simulink model "three_phase_induction_motor_speed_controller"  (R2020b)
settings: Solver=FixedStepAuto  StartTime=0.0  StopTime=200  RelTol=1e-3
undefined symbols (not defined in the file): Continuous, gcbh, J, Lm, Lr, Ls, p, Rr, Rs, sps, sps_rtmsupport, spsTriangleGeneratorModel
libraries: powerlib x13, simulink x5, pid_lib x2
settings Model: Creator=Vibhusha  LastModifiedBy=Vibhusha
settings DataIOCC: ReturnWorkspaceOutputs=off
settings DebuggingCC: ArithmeticOperatorsInVariantConditions=warning
settings SFSimCC: SimUseLocalCustomCode=off  CustomCodeUndefinedFunction=UseInterfaceOnly
settings RTWCC: RTWUseLocalCustomCode=off

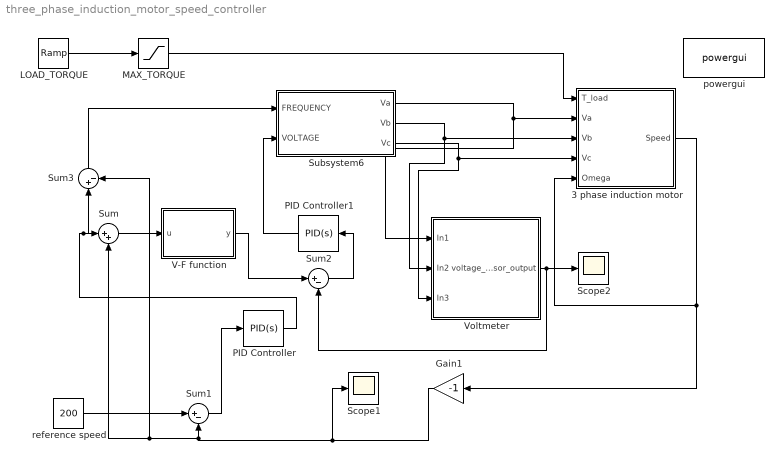
== system three_phase_induction_motor_speed_controller ==
  3 phase induction motor : Subsystem
  Gain1 : Gain  Gain=-1
  LOAD_TORQUE : simulink/Sources/Ramp  slope=0.1  start=0  InitialOutput=0
  MAX_TORQUE : Saturate  UpperLimit=5  LowerLimit=0
  PID Controller : pid_lib/PID Controller  Controller=PID  Form=Parallel  TimeDomain=Continuous-time  UseExternalTs=off  SampleTime=-1  IntegratorMethod=Forward Euler  FilterMethod=Forward Euler  ControllerParametersSource=internal  P=400  I=0.00001  D=0.0001  UseFilter=on  N=50  TunerSelectOption=Transfer Function Based (PID Tuner App)  InitialConditionSource=internal  InitialConditionForIntegrator=0  InitialConditionForFilter=0  DifferentiatorICPrevScaledInput=0  ExternalReset=none  TrackingMode=off  Kt=1  LimitOutput=on  SatLimitsSource=internal  UpperSaturationLimit=4000  LowerSaturationLimit=0  LinearizeAsGain=on  AntiWindupMode=none  Kb=1  POutMin=[]  POutMax=[]  IOutMin=[]  IOutMax=[]  DOutMin=[]  DOutMax=[]  NOutMin=[]  NOutMax=[]  SumOutMin=[]  SumOutMax=[]  SaturationOutMin=[]  SaturationOutMax=[]  PParamMin=[]  PParamMax=[]  IParamMin=[]  IParamMax=[]  DParamMin=[]  DParamMax=[]  NParamMin=[]  NParamMax=[]  KbParamMin=[]  KbParamMax=[]  KtParamMin=[]  KtParamMax=[]  KbOutMin=[]  KbOutMax=[]  KtOutMin=[]  KtOutMax=[]  IntegratorOutMin=[]  IntegratorOutMax=[]  FilterOutMin=[]  FilterOutMax=[]  SumI1OutMin=[]  SumI1OutMax=[]  SumI2OutMin=[]  SumI2OutMax=[]  SumI3OutMin=[]  SumI3OutMax=[]  SumI4OutMin=[]  SumI4OutMax=[]  SumDOutMin=[]  SumDOutMax=[]  DifferentiatorOutMin=[]  DifferentiatorOutMax=[]  FilterDiffOutCoefMin=[]  FilterDiffOutCoefMax=[]  ReciprocalOutMin=[]  ReciprocalOutMax=[]  SumDenOutMin=[]  SumDenOutMax=[]  SumNumOutMin=[]  SumNumOutMax=[]  DivideOutMin=[]  DivideOutMax=[]  UdiffTsProdOutMin=[]  UdiffTsProdOutMax=[]  NTsProdOutMin=[]  NTsProdOutMax=[]  UintegralTsProdOutMin=[]  UintegralTsProdOutMax=[]  UngainTsProdOutMin=[]  UngainTsProdOutMax=[]  IntegratorContinuousStateAttributes=''  IntegratorStateMustResolveToSignalObject=off  IntegratorRTWStateStorageClass=Auto  FilterContinuousStateAttributes=''  FilterStateMustResolveToSignalObject=off  FilterRTWStateStorageClass=Auto  ParallelPVariant=InternalParameters  IdealPVariant=Disabled  IVariant=InternalParameters  DVariant=InternalParameters  IntegratorVariant=Continuous  SatVariant=Enabled  AWVariant=Passthrough  PCopyVariant=Disabled  TRVariant=Disabled  FdbkBlocksVariant=Forward  IdealPFdbkVariant=Disabled  SatFdbkVariant=Disabled  DerivativeFilterVariant=ContFilter  NVariant=InternalParameters  NCopyVariant=Disabled  FilterICVariant=InternalICsFilter  IntegratorICVariant=InternalICs  ExternalResetVariant=Disabled  TRSumVariant=Passthrough  SumFdbkVariant=Disabled  SumVariant=Sum_PID  TsampFilterVariant=InternalTs  TsampNgainVariant=Passthrough  TsampIntegralVariant=Passthrough  ExternalSaturationOutDataTypeStr=Inherit: Same as second input
  PID Controller1 : pid_lib/PID Controller  Controller=PID  Form=Parallel  TimeDomain=Continuous-time  UseExternalTs=off  SampleTime=-1  IntegratorMethod=Forward Euler  FilterMethod=Forward Euler  ControllerParametersSource=internal  P=400  I=0.00001  D=0  UseFilter=on  N=50  TunerSelectOption=Transfer Function Based (PID Tuner App)  InitialConditionSource=internal  InitialConditionForIntegrator=0  InitialConditionForFilter=0  DifferentiatorICPrevScaledInput=0  ExternalReset=none  TrackingMode=off  Kt=1  LimitOutput=on  SatLimitsSource=internal  UpperSaturationLimit=inf  LowerSaturationLimit=1  LinearizeAsGain=on  AntiWindupMode=none  Kb=1  POutMin=[]  POutMax=[]  IOutMin=[]  IOutMax=[]  DOutMin=[]  DOutMax=[]  NOutMin=[]  NOutMax=[]  SumOutMin=[]  SumOutMax=[]  SaturationOutMin=[]  SaturationOutMax=[]  PParamMin=[]  PParamMax=[]  IParamMin=[]  IParamMax=[]  DParamMin=[]  DParamMax=[]  NParamMin=[]  NParamMax=[]  KbParamMin=[]  KbParamMax=[]  KtParamMin=[]  KtParamMax=[]  KbOutMin=[]  KbOutMax=[]  KtOutMin=[]  KtOutMax=[]  IntegratorOutMin=[]  IntegratorOutMax=[]  FilterOutMin=[]  FilterOutMax=[]  SumI1OutMin=[]  SumI1OutMax=[]  SumI2OutMin=[]  SumI2OutMax=[]  SumI3OutMin=[]  SumI3OutMax=[]  SumI4OutMin=[]  SumI4OutMax=[]  SumDOutMin=[]  SumDOutMax=[]  DifferentiatorOutMin=[]  DifferentiatorOutMax=[]  FilterDiffOutCoefMin=[]  FilterDiffOutCoefMax=[]  ReciprocalOutMin=[]  ReciprocalOutMax=[]  SumDenOutMin=[]  SumDenOutMax=[]  SumNumOutMin=[]  SumNumOutMax=[]  DivideOutMin=[]  DivideOutMax=[]  UdiffTsProdOutMin=[]  UdiffTsProdOutMax=[]  NTsProdOutMin=[]  NTsProdOutMax=[]  UintegralTsProdOutMin=[]  UintegralTsProdOutMax=[]  UngainTsProdOutMin=[]  UngainTsProdOutMax=[]  IntegratorContinuousStateAttributes=''  IntegratorStateMustResolveToSignalObject=off  IntegratorRTWStateStorageClass=Auto  FilterContinuousStateAttributes=''  FilterStateMustResolveToSignalObject=off  FilterRTWStateStorageClass=Auto  ParallelPVariant=InternalParameters  IdealPVariant=Disabled  IVariant=InternalParameters  DVariant=InternalParameters  IntegratorVariant=Continuous  SatVariant=Enabled  AWVariant=Passthrough  PCopyVariant=Disabled  TRVariant=Disabled  FdbkBlocksVariant=Forward  IdealPFdbkVariant=Disabled  SatFdbkVariant=Disabled  DerivativeFilterVariant=ContFilter  NVariant=InternalParameters  NCopyVariant=Disabled  FilterICVariant=InternalICsFilter  IntegratorICVariant=InternalICs  ExternalResetVariant=Disabled  TRSumVariant=Passthrough  SumFdbkVariant=Disabled  SumVariant=Sum_PID  TsampFilterVariant=InternalTs  TsampNgainVariant=Passthrough  TsampIntegralVariant=Passthrough  ExternalSaturationOutDataTypeStr=Inherit: Same as second input
  Scope1 : Scope
  Scope2 : Scope
  Subsystem6 : Subsystem
  Sum : Sum  Inputs=|++
  Sum1 : Sum  Inputs=|+-
  Sum2 : Sum  Inputs=|+-
  Sum3 : Sum  Inputs=|+-
  V-F function : MATLAB Function  TreatAsAtomicUnit=on
  Voltmeter : Subsystem
  powergui : powerlib/powergui  Priority=1  SimulationMode=Continuous  SampleTime=50e-6  frequency=60  Iterations=50  frequencyindice=0  Pbase=100e6  ErrMax=1e-4  UnitsV=kV  UnitsW=MW  buscounter=0  FunctionMessages=off  echomessages=off  EnableUseOfTLC=off  CurrentSourceSwitches=off  DisableSnubberDevices=off  DisableRonSwitches=off  DisableVfSwitches=off  DisplayEquations=off  AutomaticDiscreteSolvers=off  SolverType=Tustin/Backward Euler (TBE)  Interpol=off  ExternalGateDelay=off  methode=off  Ts=100  x0status=blocks  SPID=on  SwTol=0  HookPort=off  NonlinearTolerance=1e-4  nMaxIteration=100  ContinueOnMaxIteration=off  RestoreLinks=warning  ResistiveCurrentMeasurement=off  Frange=[0:2:500]  Ylog=off  Xlog=on  ShowGrid=off  save=off  variable=ZData  structure=0  ZoomFFT=off  StartTime=0.0  cycles=1  DisplayStyle=1  fundamental=60  FreqAxis=off  MaxFrequency=1000  frequencyindicesteady=1  RmsSteady=1  display=off
  reference speed : Constant  Value=200
  wires:
  Subsystem6/1(Va) -> Voltmeter/1(In1), 3 phase induction motor/2(Va)
  Subsystem6/2(Vb) -> Voltmeter/2(In2), 3 phase induction motor/3(Vb)
  Subsystem6/3(Vc) -> Voltmeter/3(In3), 3 phase induction motor/4(Vc)
  reference speed/1 -> Sum1/1
  Sum1/1 -> PID Controller/1
  Gain1/1 -> Sum3/2, Sum/2, Sum1/2, Scope1/1
  V-F function/1(y) -> Sum2/1
  Sum2/1 -> PID Controller1/1
  PID Controller1/1 -> Subsystem6/2(VOLTAGE)
  PID Controller/1 -> Sum3/1, Sum/1
  LOAD_TORQUE/1 -> MAX_TORQUE/1
  Voltmeter/1(voltage_sensor_output) -> Scope2/1, Sum2/2
  3 phase induction motor/1(Speed) -> Gain1/1, 3 phase induction motor/5(Omega)
  MAX_TORQUE/1 -> 3 phase induction motor/1(T_load)
  Sum/1 -> V-F function/1(u)
  Sum3/1 -> Subsystem6/1(FREQUENCY)

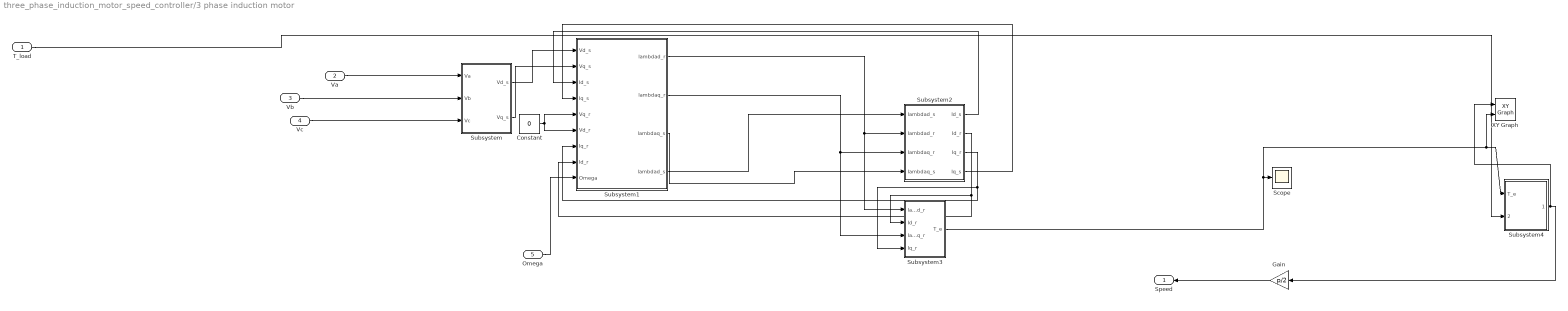
== system three_phase_induction_motor_speed_controller/3 phase induction motor ==
  T_load : Inport
  Va : Inport  Port=2
  Vb : Inport  Port=3
  Vc : Inport  Port=4
  Omega : Inport  Port=5
  Constant : Constant  Value=0
  Gain : Gain  Gain=p/2
  Scope : Scope
  Subsystem : Subsystem
  Subsystem1 : Subsystem
  Subsystem2 : Subsystem
  Subsystem3 : Subsystem
  Subsystem4 : Subsystem
  XY Graph : simulink/Sinks/XY Graph  xmin=-1  xmax=1  ymin=-1  ymax=1  st=-1
  Speed : Outport
  wires:
  Subsystem2/3(Iq_r) -> Subsystem3/4(Iq_r), Subsystem1/7(Iq_r)
  Subsystem3/1(T_e) -> XY Graph/2, Subsystem4/1(T_e), Scope/1
  Subsystem2/2(Id_r) -> Subsystem1/8(Id_r), Subsystem3/2(Id_r)
  Subsystem2/1(Id_s) -> Subsystem1/3(Id_s)
  Subsystem2/4(Iq_s) -> Subsystem1/4(Iq_s)
  Vc/1 -> Subsystem/3(Vc)
  Va/1 -> Subsystem/1(Va)
  Subsystem1/1(lambdad_r) -> Subsystem2/2(Iambdad_r), Subsystem3/1(lambdad_r)
  Subsystem1/3(lambdaq_s) -> Subsystem2/4(Iambdaq_s)
  Constant/1 -> Subsystem1/6(Vd_r), Subsystem1/5(Vq_r)
  Subsystem/2(Vq_s) -> Subsystem1/2(Vq_s)
  Omega/1 -> Subsystem1/9(Omega)
  T_load/1 -> Subsystem4/2(T_load)
  Subsystem/1(Vd_s) -> Subsystem1/1(Vd_s)
  Subsystem1/2(lambdaq_r) -> Subsystem3/3(Iambdaq_r), Subsystem2/3(Iambdaq_r)
  Subsystem4/1(W_mech) -> XY Graph/1, Gain/1
  Vb/1 -> Subsystem/2(Vb)
  Subsystem1/4(lambdad_s) -> Subsystem2/1(Iambdad_s)
  Gain/1 -> Speed/1

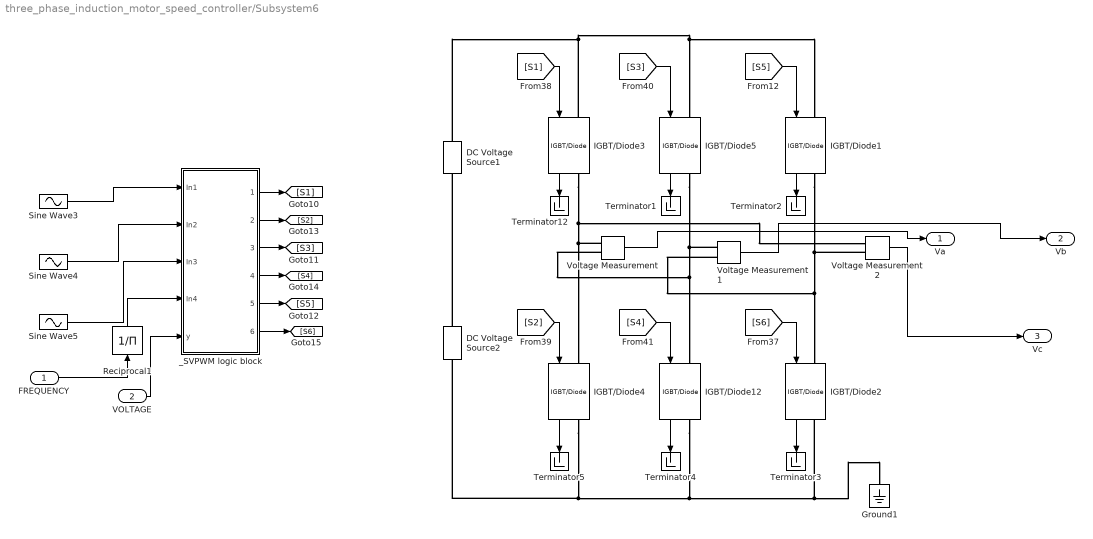
== system three_phase_induction_motor_speed_controller/Subsystem6 ==
  FREQUENCY : Inport
  VOLTAGE : Inport  Port=2
  DC Voltage Source1 : powerlib/Electrical Sources/DC Voltage Source  Amplitude=125  Measurements=None
  DC Voltage Source2 : powerlib/Electrical Sources/DC Voltage Source  Amplitude=125  Measurements=None
  Ground1 : powerlib/Elements/Ground  LConnTagsString=a
  IGBT/Diode{1..5,12} (6 alike) : powerlib/Power Electronics/IGBT//Diode  Ron=1e-3  Rs=1e5  Cs=inf  Measurements=on
  Reciprocal1 : Product  Inputs=/
  Sine Wave3 : Sin  Frequency=50*2*pi  SampleTime=0
  Sine Wave4 : Sin  Frequency=50*2*pi  Phase=pi*(-2/3)  SampleTime=0
  Sine Wave5 : Sin  Frequency=50*2*pi  Phase=pi*(2/3)  SampleTime=0
  Terminator{1..5,12} (6 alike) : Terminator
  Voltage Measurement : powerlib/Measurements/Voltage Measurement  PhasorSimulation=off  OutputType=Complex  PSBequivalent=0
  Voltage Measurement1 : powerlib/Measurements/Voltage Measurement  PhasorSimulation=off  OutputType=Complex  PSBequivalent=0
  Voltage Measurement2 : powerlib/Measurements/Voltage Measurement  PhasorSimulation=off  OutputType=Complex  PSBequivalent=0
  _SVPWM logic block : Subsystem
  Va : Outport
  Vb : Outport  Port=2
  Vc : Outport  Port=3
  wires:
  Sine Wave5/1 -> _SVPWM logic block/3(In3)
  IGBT/Diode3/1 -> Terminator12/1
  [S1] -> IGBT/Diode3/1
  _SVPWM logic block/6(6) -> [S6]
  Sine Wave4/1 -> _SVPWM logic block/2(In2)
  _SVPWM logic block/1(1) -> [S1]
  IGBT/Diode1/1 -> Terminator2/1
  IGBT/Diode2/1 -> Terminator3/1
  IGBT/Diode4/1 -> Terminator5/1
  IGBT/Diode5/1 -> Terminator1/1
  [S2] -> IGBT/Diode4/1
  _SVPWM logic block/4(4) -> [S4]
  _SVPWM logic block/5(5) -> [S5]
  [S3] -> IGBT/Diode5/1
  [S6] -> IGBT/Diode2/1
  Sine Wave3/1 -> _SVPWM logic block/1(In1)
  [S4] -> IGBT/Diode12/1
  _SVPWM logic block/3(3) -> [S3]
  [S5] -> IGBT/Diode1/1
  IGBT/Diode12/1 -> Terminator4/1
  _SVPWM logic block/2(2) -> [S2]
  Voltage Measurement/1 -> Va/1
  Voltage Measurement1/1 -> Vb/1
  Voltage Measurement2/1 -> Vc/1
  FREQUENCY/1 -> Reciprocal1/1
  VOLTAGE/1 -> _SVPWM logic block/5(y)
  Reciprocal1/1 -> _SVPWM logic block/4(In4)
  connections:
  DC Voltage Source2/RConn1 -- DC Voltage Source1/LConn1
  IGBT/Diode1/RConn1 -- Voltage Measurement1/LConn2 -- IGBT/Diode2/LConn1 -- Voltage Measurement2/LConn2
  IGBT/Diode4/RConn1 -- IGBT/Diode12/RConn1 -- Ground1/LConn1 -- IGBT/Diode2/RConn1 -- DC Voltage Source2/LConn1
  IGBT/Diode5/RConn1 -- Voltage Measurement1/LConn1 -- Voltage Measurement/LConn2 -- IGBT/Diode12/LConn1
  IGBT/Diode3/RConn1 -- IGBT/Diode4/LConn1 -- Voltage Measurement/LConn1 -- Voltage Measurement2/LConn1
  IGBT/Diode3/LConn1 -- IGBT/Diode1/LConn1 -- IGBT/Diode5/LConn1 -- DC Voltage Source1/RConn1

== system three_phase_induction_motor_speed_controller/Voltmeter ==
  In1 : Inport
  In2 : Inport  Port=2
  In3 : Inport  Port=3
  Abs : Abs
  Abs1 : Abs
  Abs2 : Abs
  Sum : Sum  Inputs=|+++
  voltage_sensor_output : Outport
  wires:
  In1/1 -> Abs2/1
  Abs2/1 -> Sum/1
  In3/1 -> Abs1/1
  Abs1/1 -> Sum/3
  In2/1 -> Abs/1
  Abs/1 -> Sum/2
  Sum/1 -> voltage_sensor_output/1

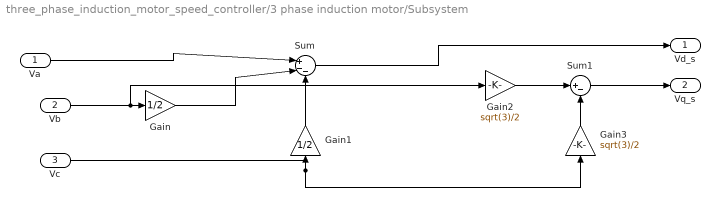
== system three_phase_induction_motor_speed_controller/3 phase induction motor/Subsystem ==
  Va : Inport
  Vb : Inport  Port=2
  Vc : Inport  Port=3
  Gain : Gain  Gain=1/2
  Gain1 : Gain  Gain=1/2
  Gain2 : Gain  Gain=sqrt(3)/2
  Gain3 : Gain  Gain=sqrt(3)/2
  Sum : Sum  Inputs=|+--
  Sum1 : Sum  Inputs=|+-
  Vd_s : Outport  VectorParamsAs1DForOutWhenUnconnected=off
  Vq_s : Outport  Port=2  VectorParamsAs1DForOutWhenUnconnected=off
  wires:
  Vc/1 -> Gain3/1, Gain1/1
  Sum1/1 -> Vq_s/1
  Vb/1 -> Gain2/1, Gain/1
  Gain2/1 -> Sum1/1
  Gain3/1 -> Sum1/2
  Gain/1 -> Sum/2
  Va/1 -> Sum/1
  Gain1/1 -> Sum/3
  Sum/1 -> Vd_s/1

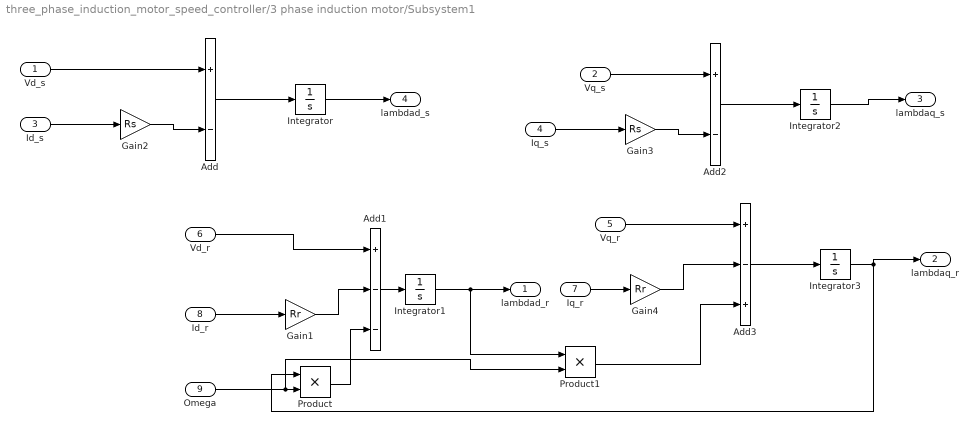
== system three_phase_induction_motor_speed_controller/3 phase induction motor/Subsystem1 ==
  Vd_s : Inport
  Vq_s : Inport  Port=2
  Id_s : Inport  Port=3
  Iq_s : Inport  Port=4
  Vq_r : Inport  Port=5
  Vd_r : Inport  Port=6
  Iq_r : Inport  Port=7
  Id_r : Inport  Port=8
  Omega : Inport  Port=9
  Add : Sum  Inputs=+-
  Add1 : Sum  Inputs=+--
  Add2 : Sum  Inputs=+-
  Add3 : Sum  Inputs=+-+
  Gain1 : Gain  Gain=Rr
  Gain2 : Gain  Gain=Rs
  Gain3 : Gain  Gain=Rs
  Gain4 : Gain  Gain=Rr
  Integrator{,1..3} (4 alike) : Integrator
  Product : Product
  Product1 : Product
  lambdad_r : Outport  VectorParamsAs1DForOutWhenUnconnected=off
  lambdaq_r : Outport  Port=2  VectorParamsAs1DForOutWhenUnconnected=off
  lambdaq_s : Outport  Port=3  VectorParamsAs1DForOutWhenUnconnected=off
  lambdad_s : Outport  Port=4  VectorParamsAs1DForOutWhenUnconnected=off
  wires:
  Integrator/1 -> lambdad_s/1
  Gain2/1 -> Add/2
  Integrator3/1 -> lambdaq_r/1, Product/1
  Vd_r/1 -> Add1/1
  Id_r/1 -> Gain1/1
  Add/1 -> Integrator/1
  Integrator2/1 -> lambdaq_s/1
  Id_s/1 -> Gain2/1
  Product/1 -> Add1/3
  Gain3/1 -> Add2/2
  Omega/1 -> Product1/2, Product/2
  Add2/1 -> Integrator2/1
  Integrator1/1 -> lambdad_r/1, Product1/1
  Gain1/1 -> Add1/2
  Vq_r/1 -> Add3/1
  Iq_r/1 -> Gain4/1
  Add1/1 -> Integrator1/1
  Vq_s/1 -> Add2/1
  Iq_s/1 -> Gain3/1
  Product1/1 -> Add3/3
  Add3/1 -> Integrator3/1
  Gain4/1 -> Add3/2
  Vd_s/1 -> Add/1

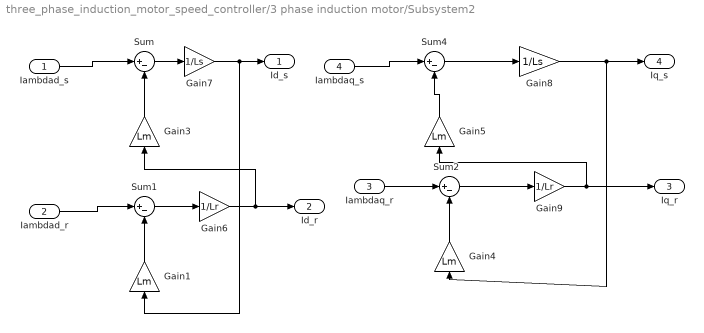
== system three_phase_induction_motor_speed_controller/3 phase induction motor/Subsystem2 ==
  Iambdad_s : Inport
  Iambdad_r : Inport  Port=2
  Iambdaq_r : Inport  Port=3
  Iambdaq_s : Inport  Port=4
  Gain{1,3..5} (4 alike) : Gain  Gain=Lm
  Gain6 : Gain  Gain=1/Lr
  Gain7 : Gain  Gain=1/Ls
  Gain8 : Gain  Gain=1/Ls
  Gain9 : Gain  Gain=1/Lr
  Sum{,1..2,4} (4 alike) : Sum  Inputs=|+-
  Id_s : Outport  VectorParamsAs1DForOutWhenUnconnected=off
  Id_r : Outport  Port=2  VectorParamsAs1DForOutWhenUnconnected=off
  Iq_r : Outport  Port=3  VectorParamsAs1DForOutWhenUnconnected=off
  Iq_s : Outport  Port=4  VectorParamsAs1DForOutWhenUnconnected=off
  wires:
  Sum/1 -> Gain7/1
  Gain6/1 -> Id_r/1, Gain3/1
  Iambdad_s/1 -> Sum/1
  Gain4/1 -> Sum2/2
  Gain8/1 -> Iq_s/1, Gain4/1
  Sum2/1 -> Gain9/1
  Gain5/1 -> Sum4/2
  Gain3/1 -> Sum/2
  Gain9/1 -> Iq_r/1, Gain5/1
  Gain7/1 -> Id_s/1, Gain1/1
  Iambdad_r/1 -> Sum1/1
  Iambdaq_r/1 -> Sum2/1
  Gain1/1 -> Sum1/2
  Sum1/1 -> Gain6/1
  Sum4/1 -> Gain8/1
  Iambdaq_s/1 -> Sum4/1

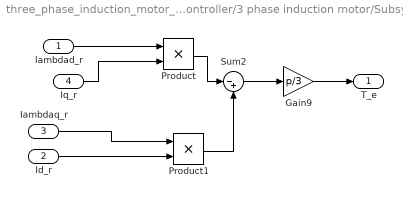
== system three_phase_induction_motor_speed_controller/3 phase induction motor/Subsystem3 ==
  lambdad_r : Inport
  Id_r : Inport  Port=2
  Iambdaq_r : Inport  Port=3
  Iq_r : Inport  Port=4
  Gain9 : Gain  Gain=p/3
  Product : Product
  Product1 : Product
  Sum2 : Sum  Inputs=|-+
  T_e : Outport  VectorParamsAs1DForOutWhenUnconnected=off
  wires:
  Product1/1 -> Sum2/2
  Product/1 -> Sum2/1
  Sum2/1 -> Gain9/1
  Gain9/1 -> T_e/1
  Iambdaq_r/1 -> Product1/1
  Iq_r/1 -> Product/2
  lambdad_r/1 -> Product/1
  Id_r/1 -> Product1/2

== system three_phase_induction_motor_speed_controller/3 phase induction motor/Subsystem4 ==
  T_e : Inport
  T_load : Inport  Port=2
  Gain : Gain  Gain=1/J
  Gain1 : Gain  Gain=2/p
  Integrator : Integrator
  Sum : Sum  Inputs=|+-
  W_mech : Outport  VectorParamsAs1DForOutWhenUnconnected=off
  wires:
  Sum/1 -> Gain/1
  T_load/1 -> Sum/2
  Integrator/1 -> Gain1/1
  Gain/1 -> Integrator/1
  Gain1/1 -> W_mech/1
  T_e/1 -> Sum/1

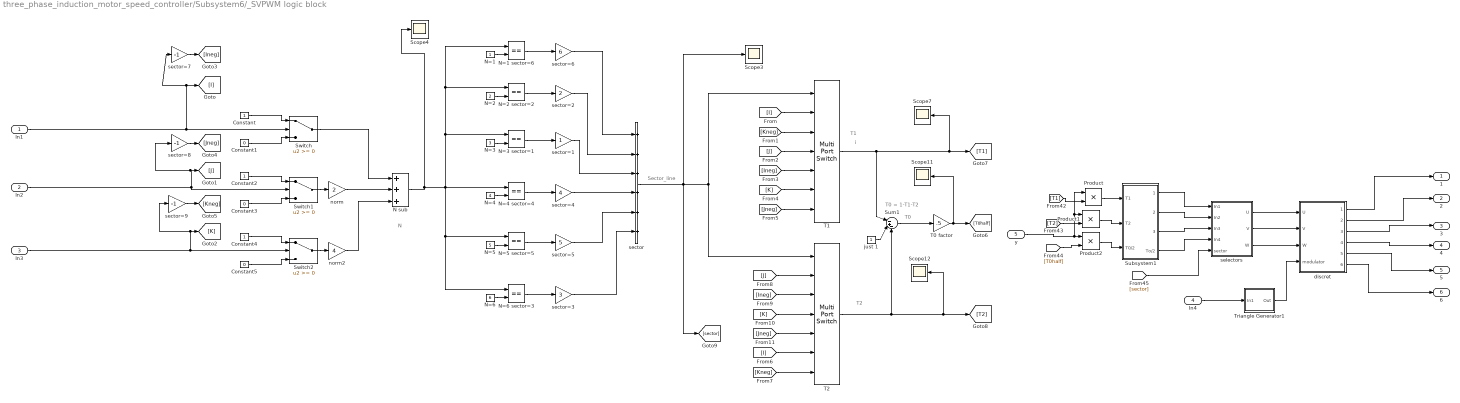
== system three_phase_induction_motor_speed_controller/Subsystem6/_SVPWM logic block ==
  note: T0
  note: T0 = 1-T1-T2
  note: T2
  note: T1
  note: i
  note: Sector_line
  note: N
  In1 : Inport
  In2 : Inport  Port=2
  In3 : Inport  Port=3
  In4 : Inport  Port=4
  y : Inport  Port=5
  Constant : Constant
  Constant1 : Constant  Value=0
  Constant2 : Constant
  Constant3 : Constant  Value=0
  Constant4 : Constant
  Constant5 : Constant  Value=0
  N sub : Sum  Inputs=+++
  N=1 : Constant
  N=1 sector=6 : RelationalOperator  Operator===  OutDataTypeStr=boolean  RndMeth=Nearest
  N=2 : Constant  Value=2
  N=2 sector=2 : RelationalOperator  Operator===  OutDataTypeStr=boolean  RndMeth=Nearest
  N=3 : Constant  Value=3
  N=3 sector=1 : RelationalOperator  Operator===  OutDataTypeStr=boolean  RndMeth=Nearest
  N=4 : Constant  Value=4
  N=4 sector=4 : RelationalOperator  Operator===  OutDataTypeStr=boolean  RndMeth=Nearest
  N=5 : Constant  Value=5
  N=5 sector=5 : RelationalOperator  Operator===  OutDataTypeStr=boolean  RndMeth=Nearest
  N=6 : Constant  Value=6
  N=6 sector=3 : RelationalOperator  Operator===  OutDataTypeStr=boolean  RndMeth=Nearest
  Product : Product
  Product1 : Product
  Product2 : Product
  Scope{3..4,7,11..12} (5 alike) : Scope
  Subsystem1 : Subsystem
  Sum1 : Sum  Inputs=|-+-
  Switch : Switch
  Switch1 : Switch
  Switch2 : Switch
  T0 factor : Gain  Gain=.5
  T1 : MultiPortSwitch  DataPortOrder=Specify indices  Inputs=4  DataPortIndices={1,2,3,4,5,6}
  T2 : MultiPortSwitch  DataPortOrder=Specify indices  Inputs=4  DataPortIndices={1,2,3,4,5,6}
  Triangle Generator1 : Subsystem  AncestorBlock=|  DialogController=POWERSYS.PowerSysDialog  LoadFcn=sps_rtmsupport('LoadFcn', gcbh);  StartFcn=sps_rtmsupport('StartFcn', gcbh);  StopFcn=sps_rtmsupport('StopFcn', gcbh);  mask(Triangle Generator){Freq=100, Phase=180, Ts=0}
      | powerlib_meascontrol/Pulse & Signal
      | Generators/Triangle
      | Generator
      mask prompts: Freq "Frequency (Hz):"; Phase "Phase (degrees):"; Ts "Sample time:"
      mask help: Generate a symmetrical triangle wave with peak amplitude of +/- 1.
      mask init:
      | block = gcb;
      | [WantBlockChoice,Ts,sps] = powericon('TriangleGeneratorInit',block,Phase,Freq,Ts);
      | powericon('SetInternalModels','set',block,WantBlockChoice);
      settings: CopyFcn=sps_rtmsupport('CopyFcn', gcbh);  DeleteFcn=sps_rtmsupport('DeleteFcn', gcbh);  UndoDeleteFcn=sps_rtmsupport('UndoDeleteFcn', gcbh);  ModelCloseFcn=sps_rtmsupport('ModelCloseFcn', gcbh);  PreSaveFcn=sps_rtmsupport('PreSaveFcn', gcbh);  PostSaveFcn=sps_rtmsupport('PostSaveFcn', gcbh);  NameChangeFcn=sps_rtmsupport('NameChangeFcn', gcbh);  PreCopyFcn=sps_rtmsupport('PreCopyFcn', gcbh);  OpenFcn=sps_rtmsupport('OpenFcn', gcbh, []);  CloseFcn=sps_rtmsupport('CloseFcn', gcbh);  PreDeleteFcn=sps_rtmsupport('PreDeleteFcn', gcbh);
      mask Help: helpview(psbhelp);
      mask Display: plot([sps.time sps.time+sps.time(end)],repmat(sps.Out,1,2))
  discret : Subsystem
  just 1 : Constant
  norm : Gain  Gain=2
  norm2 : Gain  Gain=4
  sector : Sum  Inputs=++++++
  sector=1 : Gain
  sector=2 : Gain  Gain=2
  sector=3 : Gain  Gain=3
  sector=4 : Gain  Gain=4
  sector=5 : Gain  Gain=5
  sector=6 : Gain  Gain=6
  sector=7 : Gain  Gain=-1
  sector=8 : Gain  Gain=-1
  sector=9 : Gain  Gain=-1
  selectors : Subsystem
  1 : Outport
  2 : Outport  Port=2
  3 : Outport  Port=3
  4 : Outport  Port=4
  5 : Outport  Port=5
  6 : Outport  Port=6
  wires:
  Constant1/1 -> Switch/3
  In1/1 -> Switch/2, sector=7/1, [I]
  Constant2/1 -> Switch1/1
  Constant/1 -> Switch/1
  Constant3/1 -> Switch1/3
  N=1/1 -> N=1 sector=6/2
  N=6/1 -> N=6 sector=3/2
  N=6 sector=3/1 -> sector=3/1
  N=5/1 -> N=5 sector=5/2
  N sub/1 -> Scope4/1, N=6 sector=3/1, N=5 sector=5/1, N=4 sector=4/1, N=3 sector=1/1, N=2 sector=2/1, N=1 sector=6/1
  N=3 sector=1/1 -> sector=1/1
  N=3/1 -> N=3 sector=1/2
  Constant4/1 -> Switch2/1
  Switch/1 -> N sub/1
  In2/1 -> Switch1/2, [J], sector=8/1
  N=4/1 -> N=4 sector=4/2
  N=5 sector=5/1 -> sector=5/1
  Switch2/1 -> norm2/1
  N=2/1 -> N=2 sector=2/2
  sector=2/1 -> sector/2
  N=2 sector=2/1 -> sector=2/1
  sector=4/1 -> sector/4
  sector=5/1 -> sector/5
  N=4 sector=4/1 -> sector=4/1
  sector=1/1 -> sector/3
  Switch1/1 -> norm/1
  sector=3/1 -> sector/6
  N=1 sector=6/1 -> sector=6/1
  sector=6/1 -> sector/1
  In3/1 -> Switch2/2, sector=9/1, [K]
  Constant5/1 -> Switch2/3
  [I] -> T1/2
  [Kneg] -> T2/7
  sector=8/1 -> [Jneg]
  Sum1/1 -> T0 factor/1
  T0 factor/1 -> Scope11/1, [T0half]
  sector/1 -> [sector], Scope3/1, T2/1, T1/1
  [Ineg] -> T1/5
  sector=7/1 -> [Ineg]
  norm2/1 -> N sub/3
  [Jneg] -> T1/7
  [J] -> T2/2
  [K] -> T1/6
  [J] -> T1/4
  [I] -> T2/6
  [K] -> T2/4
  T1/1 -> Scope7/1, [T1], Sum1/1
  sector=9/1 -> [Kneg]
  just 1/1 -> Sum1/2
  [Kneg] -> T1/3
  [Jneg] -> T2/5
  norm/1 -> N sub/2
  [Ineg] -> T2/3
  selectors/3(W) -> discret/3(W)
  Triangle Generator1/1(Out) -> discret/4(modulator)
  discret/2(2) -> 2/1
  discret/3(3) -> 3/1
  Subsystem1/2(T1+To/2) -> selectors/2(In2)
  discret/4(4) -> 4/1
  Subsystem1/1(T1+T2+To/2) -> selectors/1(In1)
  [T1] -> Product/2
  discret/1(1) -> 1/1
  T2/1 -> Sum1/3, Scope12/1, [T2]
  selectors/2(V) -> discret/2(V)
  Subsystem1/4(To/2) -> selectors/4(In4)
  [sector] -> selectors/5("sector ")
  Subsystem1/3(T2+To/2) -> selectors/3(In3)
  selectors/1(U) -> discret/1(U)
  discret/5(5) -> 5/1
  discret/6(6) -> 6/1
  In4/1 -> Triangle Generator1/1(In1)
  [T2] -> Product1/2
  Product/1 -> Subsystem1/1(T1)
  [T0half] -> Product2/2
  Product1/1 -> Subsystem1/2(T2)
  Product2/1 -> Subsystem1/3(T0/2)
  y/1 -> Product1/1, Product/1, Product2/1

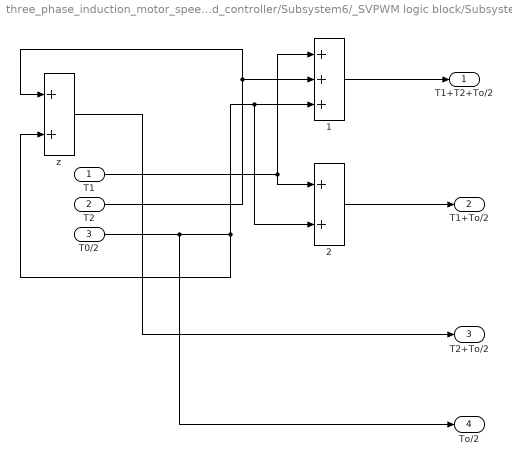
== system three_phase_induction_motor_speed_controller/Subsystem6/_SVPWM logic block/Subsystem1 ==
  T1 : Inport
  T2 : Inport  Port=2
  T0/2 : Inport  Port=3
  1 : Sum  Inputs=+++
  2 : Sum
  z : Sum
  T1+T2+To/2 : Outport
  T1+To/2 : Outport  Port=2
  T2+To/2 : Outport  Port=3
  To/2 : Outport  Port=4
  wires:
  T1/1 -> 2/1, 1/1
  T0/2/1 -> z/2, 1/3, 2/2, To/2/1
  2/1 -> T1+To/2/1
  1/1 -> T1+T2+To/2/1
  T2/1 -> z/1, 1/2
  z/1 -> T2+To/2/1

== system three_phase_induction_motor_speed_controller/Subsystem6/_SVPWM logic block/Triangle Generator1 ==
  In1 : Inport
  Model : Subsystem  AncestorBlock=spsTriangleGeneratorModel/Continuous
  Out : Outport  VectorParamsAs1DForOutWhenUnconnected=off
  wires:
  Model/1(Out) -> Out/1
  In1/1 -> Model/1(In1)

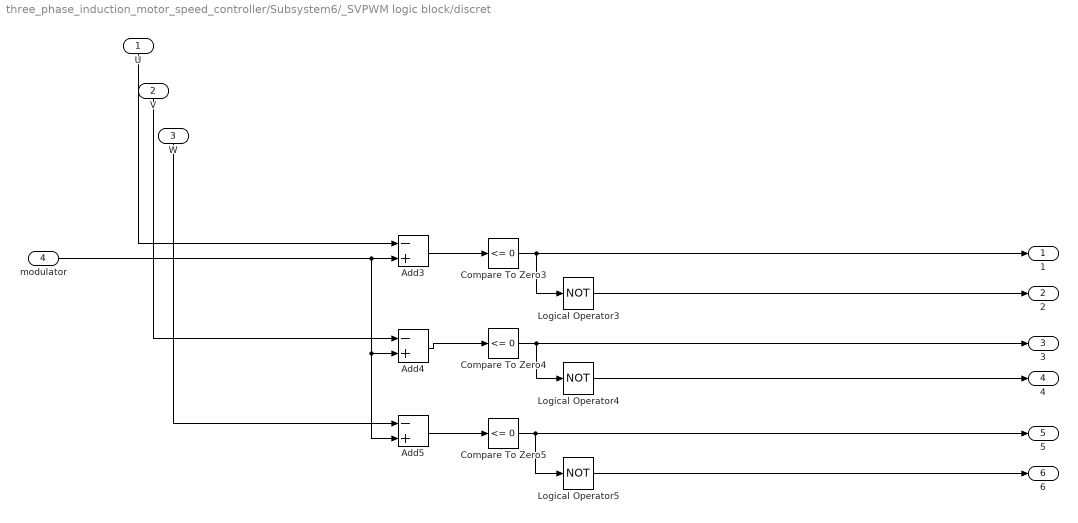
== system three_phase_induction_motor_speed_controller/Subsystem6/_SVPWM logic block/discret ==
  U : Inport
  V : Inport  Port=2
  W : Inport  Port=3
  modulator : Inport  Port=4
  Add3 : Sum  Inputs=-+
  Add4 : Sum  Inputs=-+
  Add5 : Sum  Inputs=-+
  Compare To Zero3 : simulink/Logic and Bit Operations/Compare To Zero  relop=<=  OutDataTypeStr=boolean
  Compare To Zero4 : simulink/Logic and Bit Operations/Compare To Zero  relop=<=  OutDataTypeStr=boolean
  Compare To Zero5 : simulink/Logic and Bit Operations/Compare To Zero  relop=<=  OutDataTypeStr=boolean
  Logical Operator3 : Logic  Operator=NOT  AllPortsSameDT=off  OutDataTypeStr=boolean
  Logical Operator4 : Logic  Operator=NOT  AllPortsSameDT=off  OutDataTypeStr=boolean
  Logical Operator5 : Logic  Operator=NOT  AllPortsSameDT=off  OutDataTypeStr=boolean
  1 : Outport
  2 : Outport  Port=2
  3 : Outport  Port=3
  4 : Outport  Port=4
  5 : Outport  Port=5
  6 : Outport  Port=6
  wires:
  Compare To Zero4/1 -> Logical Operator4/1, 3/1
  Compare To Zero5/1 -> Logical Operator5/1, 5/1
  Logical Operator3/1 -> 2/1
  Compare To Zero3/1 -> Logical Operator3/1, 1/1
  Logical Operator4/1 -> 4/1
  Logical Operator5/1 -> 6/1
  V/1 -> Add4/1
  W/1 -> Add5/1
  U/1 -> Add3/1
  Add5/1 -> Compare To Zero5/1
  Add3/1 -> Compare To Zero3/1
  Add4/1 -> Compare To Zero4/1
  modulator/1 -> Add3/2, Add5/2, Add4/2

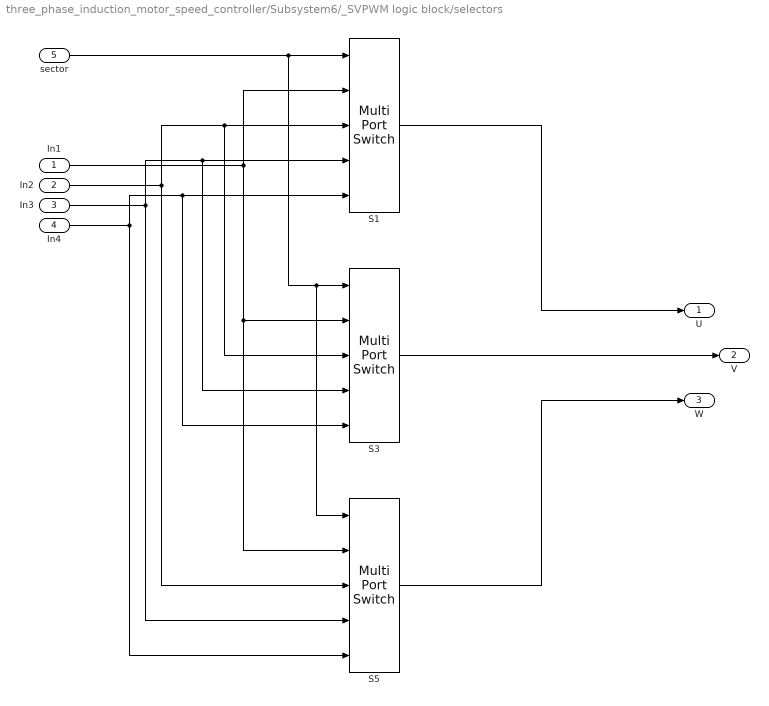
== system three_phase_induction_motor_speed_controller/Subsystem6/_SVPWM logic block/selectors ==
  In1 : Inport
  In2 : Inport  Port=2
  In3 : Inport  Port=3
  In4 : Inport  Port=4
  "sector " : Inport  Port=5
  S1 : MultiPortSwitch  DataPortOrder=Specify indices  Inputs=4  DataPortIndices={[1,6],2,5,[3,4]}
  S3 : MultiPortSwitch  DataPortOrder=Specify indices  Inputs=4  DataPortIndices={[2,3],4,1,[5,6]}
  S5 : MultiPortSwitch  DataPortOrder=Specify indices  Inputs=4  DataPortIndices={[4,5],6,3,[1,2]}
  U : Outport
  V : Outport  Port=2
  W : Outport  Port=3
  wires:
  S1/1 -> U/1
  In4/1 -> S5/5, S1/5, S3/5
  In1/1 -> S3/2, S5/2, S1/2
  In2/1 -> S5/3, S1/3, S3/3
  S5/1 -> W/1
  In3/1 -> S5/4, S1/4, S3/4
  S3/1 -> V/1
  "sector "/1 -> S5/1, S3/1, S1/1

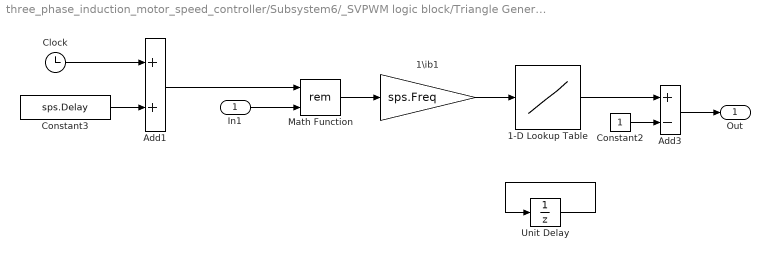
== system three_phase_induction_motor_speed_controller/Subsystem6/_SVPWM logic block/Triangle Generator1/Model ==
  In1 : Inport
  1-D Lookup Table : Lookup_n-D  NumberOfTableDimensions=1  BreakpointsForDimension1=[0 .5 1]  BeginIndexSearchUsingPreviousIndexResult=on  Table=[0 2 0]  InternalRulePriority=Speed  RndMeth=Simplest  InputSameDT=on
  1\ib1 : Gain  Gain=sps.Freq  SaturateOnIntegerOverflow=on  OutDataTypeStr=Inherit: Same as input  ParamDataTypeStr=Inherit: Same as input
  Add1 : Sum
  Add3 : Sum  Inputs=+-
  Clock : Clock
  Constant2 : Constant  SampleTime=0
  Constant3 : Constant  Value=sps.Delay  SampleTime=0
  Math Function : Math  Operator=rem  SignedPower=on  SaturateOnIntegerOverflow=on
  Unit Delay : UnitDelay  SampleTime=sps.TimeStepZ  HasFrameUpgradeWarning=on
  Out : Outport
  wires:
  1\ib1/1 -> 1-D Lookup Table/1
  Add3/1 -> Out/1
  Math Function/1 -> 1\ib1/1
  Clock/1 -> Add1/1
  In1/1 -> Math Function/2
  Constant3/1 -> Add1/2
  Unit Delay/1 -> Unit Delay/1
  Add1/1 -> Math Function/1
  1-D Lookup Table/1 -> Add3/1
  Constant2/1 -> Add3/2

== matlab function three_phase_induction_motor_speed_controller/V-F function ==
  data: u input; y output
function y = fcn(u)
    if u<1500
        y = 200+0.15*u;
        
    else
            y=400;
            
    end
